simulink model "LabControlCorrienteYPosicionCopy"  (R2023b)
settings: Solver=FixedStepAuto  StartTime=0.0  StopTime=inf  FixedStep=0.0005  RelTol=1e-3  EnableMultiTasking=on
undefined symbols (not defined in the file or in its folder): DiscIntNeverNeededParam
libraries: arduinolib x5, simulink x5, arduinosensorlib x1
settings Model: ExtModeTrigDuration=2  Creator=andre  LastModifiedBy=marti
settings OptimizationCC: EnhancedBackFolding=on  PassReuseOutputArgsAs=Individual arguments  ZeroExternalMemoryAtStartup=off  ZeroInternalMemoryAtStartup=off  MaxStackSize=64  OptimizeBlockOrder=speed  DifferentSizesBufferReuse=on  OptimizationCustomize=off  EfficientTunableParamExpr=on
settings DebuggingCC: ParameterTunabilityLossMsg=error
settings HardwareCC: ProdBitPerInt=16  ProdBitPerPointer=16  ProdBitPerSizeT=16  ProdBitPerPtrDiffT=16  ProdLargestAtomicFloat=None  ProdWordSize=8  ProdHWDeviceType=Atmel->AVR
settings SFSimCC: MATLABDynamicMemAlloc=off
settings RTWCC: Description=Embedded Coder  SystemTargetFile=ert.tlc  HardwareBoard=Arduino Mega 2560  TemplateMakefile=ert_default_tmf  Toolchain=Arduino AVR  BuildConfiguration=Faster Runs
settings CodeAppCC: ForceParamTrailComments=on  IgnoreCustomStorageClasses=off  OperatorAnnotations=on  SimulinkDataObjDesc=on  SFDataObjDesc=on  InsertBlockDesc=on
settings ERTTargetCC: SupportContinuousTime=on  SupportVariableSizeSignals=on  ExtMode=on  ExtModeTransport=3  ExtModeStaticAlloc=on  ExtModeAutomaticAllocSize=off  ExtModeStaticAllocSize=2048  ExtModeMexFile=ext_xcp  ExtModeMexArgs=0 3 115200  ExtModeIntrfLevel=Level2 - Open

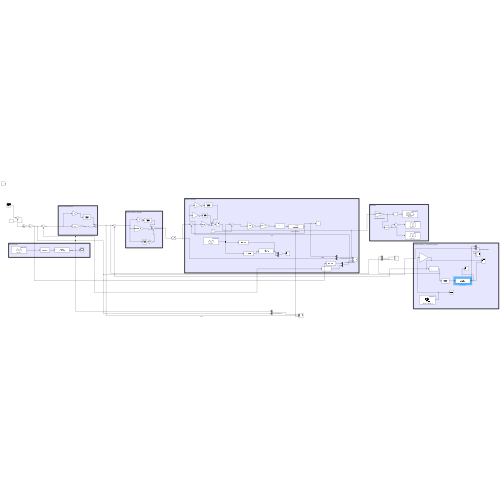
[thumbnail: Simulink's stored preview of the top-level diagram]
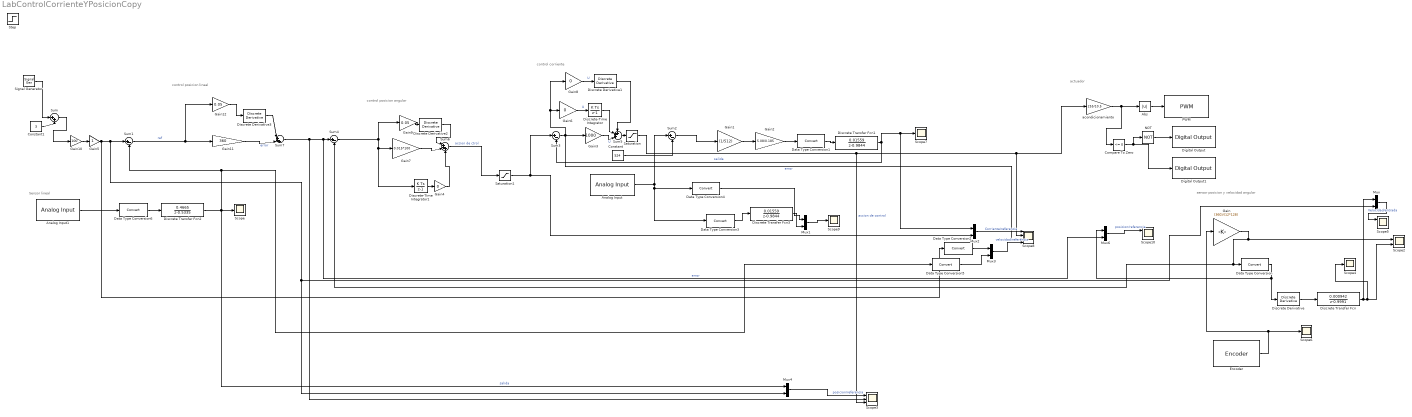
== system LabControlCorrienteYPosicionCopy ==
  note: sensor posicion y velocidad angular
  note: actuador
  note: Sensor lineal
  note: control posicion lineal
  note: control posicion angular
  note: control corriente
  Abs : Abs  SaturateOnIntegerOverflow=off
  Analog Input : arduinolib/Analog Input  pinNumber=4  ReadResultsOnly=off  ConversionTriggerSource=Software  ExternalTriggerType=uint32( 0 )  OutputDataType=uint16  EnableConversionCompleteNotify=off  EnableOuputStatus=off  SampleTime=-1  blockPlatform=arduino
  Analog Input1 : arduinolib/Analog Input  pinNumber=3  ReadResultsOnly=off  ConversionTriggerSource=Software  ExternalTriggerType=uint32( 0 )  OutputDataType=uint16  EnableConversionCompleteNotify=off  EnableOuputStatus=off  SampleTime=-1  blockPlatform=arduino
  Compare To Zero : simulink/Logic and Bit Operations/Compare To Zero  relop=<=  OutDataTypeStr=boolean
  Constant : Constant  Value=524
  Constant1 : Constant  Value=3
  Data Type Conversion{,1..6} (7 alike) : DataTypeConversion  SaturateOnIntegerOverflow=off  RndMeth=Floor
  Digital Output : arduinolib/Digital Output  pinNumber=11  Direction=output  blockPlatform=arduino
  Digital Output1 : arduinolib/Digital Output  pinNumber=10  Direction=output  blockPlatform=arduino
  Discrete Transfer Fcn : DiscreteTransferFcn  Numerator=[0.000942]  Denominator=[1 -0.9991]
  Discrete Transfer Fcn1 : DiscreteTransferFcn  Numerator=[0.01559]  Denominator=[1 -0.9844]
  Discrete Transfer Fcn2 : DiscreteTransferFcn  Numerator=[0.4665]  Denominator=[1 -0.5335]
  Discrete Transfer Fcn3 : DiscreteTransferFcn  Numerator=[0.01559]  Denominator=[1 -0.9844]
  Discrete Derivative : simulink/Quick Insert/Discrete/Discrete Derivative  gainval=1.0  ICPrevScaledInput=0.0  OutMin=[]  OutMax=[]  OutDataType=fixdt(1, 16)  OutScaling=2^-10  DoSatur=off
  Discrete Derivative1 : simulink/Discrete/Discrete Derivative  gainval=1.0  ICPrevScaledInput=0.0  OutMin=[]  OutMax=[]  OutDataType=fixdt(1, 16)  OutScaling=2^-10  DoSatur=off
  Discrete Derivative2 : simulink/Discrete/Discrete Derivative  gainval=1.0  ICPrevScaledInput=0.0  OutMin=[]  OutMax=[]  OutDataType=fixdt(1, 16)  OutScaling=2^-10  DoSatur=off
  Discrete Derivative3 : simulink/Discrete/Discrete Derivative  gainval=1.0  ICPrevScaledInput=0.0  OutMin=[]  OutMax=[]  OutDataType=fixdt(1, 16)  OutScaling=2^-10  DoSatur=off
  Discrete-Time Integrator : DiscreteIntegrator  SampleTime=-1  ICPrevOutput=DiscIntNeverNeededParam  ICPrevScaledInput=DiscIntNeverNeededParam
  Discrete-Time Integrator1 : DiscreteIntegrator  SampleTime=-1  ICPrevOutput=DiscIntNeverNeededParam  ICPrevScaledInput=DiscIntNeverNeededParam
  Encoder : arduinosensorlib/Encoder  InputA=2  InputB=3  Mode=No reset  SampleTime=-1
  Gain : Gain  Gain=(360)/(12*128)
  Gain1 : Gain  Gain=(1/512)
  Gain10 : Gain  Gain=100
  Gain11 : Gain  Gain=360
  Gain12 : Gain  Gain=0.05
  Gain2 : Gain  Gain=5.08/0.185
  Gain3 : Gain  Gain=1000
  Gain4 : Gain  Gain=0
  Gain5 : Gain
  Gain6 : Gain  Gain=0
  Gain7 : Gain  Gain=0.015*100
  Gain8 : Gain  Gain=0
  Gain9 : Gain  Gain=0.05
  Mux{,1..4,6} (6 alike) : Mux  Inputs=2
  NOT : Logic  Operator=NOT  IconShape=distinctive  AllPortsSameDT=off  OutDataTypeStr=boolean
  PWM : arduinolib/PWM  pinNumber=5  frequencyType=Default  desiredFrequency=490.2  achievableFrequency=490.2
  Saturation : Saturate  UpperLimit=10.5  LowerLimit=-10.5
  Saturation1 : Saturate  UpperLimit=3  LowerLimit=-3
  Scope{,4,6..7,9} (5 alike) : Scope
  Scope10 : Scope  NumInputPorts=3
  Scope2 : Scope  NumInputPorts=2
  Scope3 : Scope  NumInputPorts=3
  Scope5 : Scope  NumInputPorts=3
  Scope8 : Scope  NumInputPorts=4
  Signal Generator : SignalGenerator  WaveForm=square  Frequency=0.2
  Step : Step  SampleTime=0
  Sum : Sum  Inputs=|++
  Sum{1..4} (4 alike) : Sum  Inputs=|+-
  Sum5 : Sum  Inputs=+++|
  Sum6 : Sum  Inputs=|+++
  Sum7 : Sum  Inputs=|+++
  acondicionamiento : Gain  Gain=255/10.5
  wires:
  Encoder/1 -> Gain/1, Scope6/1
  Discrete Derivative/1 -> Discrete Transfer Fcn/1
  Abs/1 -> PWM/1
  Compare To Zero/1 -> NOT/1, Digital Output1/1
  NOT/1 -> Digital Output/1
  acondicionamiento/1 -> Compare To Zero/1, Abs/1
  Mux/1 -> Scope5/1  "Velocidad/entrada"
  Data Type Conversion/1 -> Mux6/1, Discrete Derivative/1
  Sum1/1 -> Gain12/1, Gain11/1  "ref"
  Gain5/1 -> Data Type Conversion2/1, Sum1/1, Mux/2, Mux4/2
  Sum6/1 -> Saturation1/1  "accion de ctrol"
  Discrete-Time Integrator1/1 -> Gain4/1
  Gain4/1 -> Sum6/3
  Gain7/1 -> Sum6/2
  Gain8/1 -> Discrete Derivative1/1  "U"
  Discrete Derivative1/1 -> Sum5/1
  Gain6/1 -> Discrete-Time Integrator/1  "U"
  Discrete-Time Integrator/1 -> Sum5/2
  Discrete Transfer Fcn/1 -> Scope4/1, Scope2/2, Mux/1
  Mux3/1 -> Scope8/4  "velocidad/referencia"
  Gain3/1 -> Sum5/3  "U"
  Mux2/1 -> Scope8/1  "Corriente/referencia"
  Data Type Conversion2/1 -> Mux3/1
  Gain2/1 -> Data Type Conversion1/1
  Data Type Conversion4/1 -> Mux1/1
  Discrete Transfer Fcn3/1 -> Mux1/2
  Mux1/1 -> Scope9/1
  Data Type Conversion1/1 -> Discrete Transfer Fcn1/1
  Sum2/1 -> Gain1/1
  Saturation/1 -> Scope3/3, acondicionamiento/1, Scope8/2  "accion de control"
  Gain1/1 -> Gain2/1
  Sum3/1 -> Gain8/1, Gain6/1, Gain3/1, Scope8/3  "error"
  Data Type Conversion3/1 -> Discrete Transfer Fcn3/1
  Discrete Transfer Fcn1/1 -> Mux2/1, Scope7/1, Sum3/2  "salida"
  Sum5/1 -> Saturation/1
  Data Type Conversion5/1 -> Mux3/2
  Analog Input/1 -> Data Type Conversion3/1, Data Type Conversion4/1, Sum2/1
  Saturation1/1 -> Mux2/2, Sum3/1
  Constant/1 -> Sum2/2
  Data Type Conversion6/1 -> Discrete Transfer Fcn2/1
  Discrete Transfer Fcn2/1 -> Sum1/2, Data Type Conversion5/1, Mux4/1, Scope/1  "salida"
  Analog Input1/1 -> Data Type Conversion6/1
  Gain9/1 -> Discrete Derivative2/1
  Discrete Derivative2/1 -> Sum6/1
  Gain10/1 -> Gain5/1
  Sum/1 -> Gain10/1
  Signal Generator/1 -> Sum/1
  Constant1/1 -> Sum/2
  Sum4/1 -> Discrete-Time Integrator1/1, Gain7/1, Gain9/1
  Sum7/1 -> Scope3/2, Mux6/2, Sum4/1  "error"
  Mux4/1 -> Scope3/1  "posicion/referencia"
  Gain/1 -> Sum4/2, Data Type Conversion/1, Scope2/1
  Mux6/1 -> Scope10/1  "posicion/referencia"
  Gain12/1 -> Discrete Derivative3/1
  Discrete Derivative3/1 -> Sum7/1
  Gain11/1 -> Sum7/2  "error"
